simulink model "LineFollowerCar"  (R2022a)
settings: Solver=VariableStepAuto  StartTime=0.0  StopTime=10.0  RelTol=1e-3
libraries: arduinolib x8, simulink x3, slpidlib x1
settings Model: Creator=shuva  LastModifiedBy=shuva

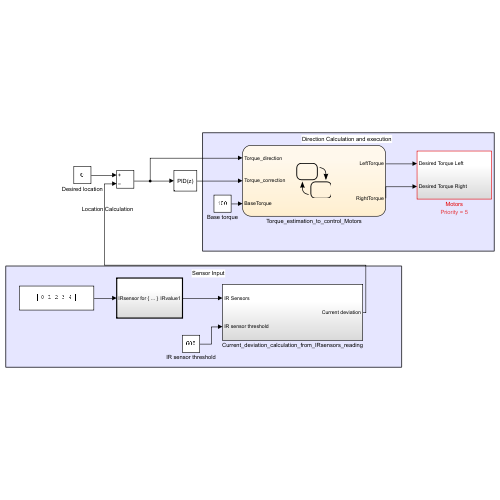
[thumbnail: Simulink's stored preview of the top-level diagram]
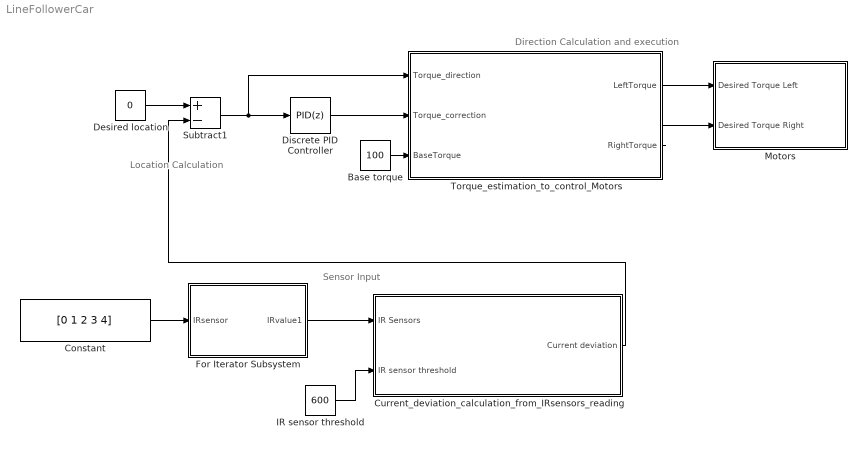
== system LineFollowerCar ==
  note: Sensor Input
  note: Direction Calculation and execution
  note: Location Calculation
  Base torque : Constant  Value=100  OutDataTypeStr=int16
  Constant : Constant  Value=[0 1 2 3 4]  OutDataTypeStr=uint8  SampleTime=0.002
  Current_deviation_calculation_from_IRsensors_reading : Subsystem
  Desired location : Constant  Value=0  OutDataTypeStr=int8
  Discrete PID Controller : slpidlib/PID Controller  Controller=PID  Form=Parallel  TimeDomain=Discrete-time  UseExternalTs=off  SampleTime=-1  IntegratorMethod=Forward Euler  FilterMethod=Forward Euler  ControllerParametersSource=internal  P=35  I=15  UseKiTs=off  D=0.005  N=60  UseFilter=off  TunerSelectOption=Transfer Function Based (PID Tuner App)  InitialConditionSource=internal  InitialConditionForIntegrator=0  InitialConditionForFilter=0  DifferentiatorICPrevScaledInput=0  ExternalReset=none  TrackingMode=off  Kt=1  LimitOutput=off  SatLimitsSource=internal  UpperSaturationLimit=inf  LowerSaturationLimit=-inf  LinearizeAsGain=on  AntiWindupMode=none  Kb=1  RndMeth=Round  PGainOutDataTypeStr=int16  PProdOutDataTypeStr=int16  POutMin=[]  POutMax=[]  IGainOutDataTypeStr=int16  IProdOutDataTypeStr=int16  IOutMin=[]  IOutMax=[]  DGainOutDataTypeStr=int16  DProdOutDataTypeStr=int16  DOutMin=[]  DOutMax=[]  NGainOutDataTypeStr=int8  NProdOutDataTypeStr=int8  NOutMin=[]  NOutMax=[]  SumOutDataTypeStr=int16  SumOutMin=[]  SumOutMax=[]  SaturationOutMin=[]  SaturationOutMax=[]  PParamDataTypeStr=int16  PParamMin=[]  PParamMax=[]  IParamDataTypeStr=int16  IParamMin=[]  IParamMax=[]  DParamDataTypeStr=int16  DParamMin=[]  DParamMax=[]  NParamDataTypeStr=int8  NParamMin=[]  NParamMax=[]  KbParamMin=[]  KbParamMax=[]  KtParamMin=[]  KtParamMax=[]  KbOutMin=[]  KbOutMax=[]  KtOutMin=[]  KtOutMax=[]  IntegratorOutDataTypeStr=int16  IntegratorOutMin=[]  IntegratorOutMax=[]  FilterOutDataTypeStr=int8  FilterOutMin=[]  FilterOutMax=[]  SumI1OutMin=[]  SumI1OutMax=[]  SumI2OutMin=[]  SumI2OutMax=[]  SumI3OutMin=[]  SumI3OutMax=[]  SumI4OutMin=[]  SumI4OutMax=[]  SumDOutDataTypeStr=int8  SumDOutMin=[]  SumDOutMax=[]  SumAccumDataTypeStr=int16  SumDAccumDataTypeStr=int8  DifferentiatorOutMin=[]  DifferentiatorOutMax=[]  FilterDiffOutCoefMin=[]  FilterDiffOutCoefMax=[]  ReciprocalOutMin=[]  ReciprocalOutMax=[]  SumDenOutMin=[]  SumDenOutMax=[]  SumNumOutMin=[]  SumNumOutMax=[]  DivideOutMin=[]  DivideOutMax=[]  UdiffTsProdOutMin=[]  UdiffTsProdOutMax=[]  NTsProdOutMin=[]  NTsProdOutMax=[]  UintegralTsProdOutMin=[]  UintegralTsProdOutMax=[]  UngainTsProdOutMin=[]  UngainTsProdOutMax=[]  IntegratorContinuousStateAttributes=''  IntegratorStateMustResolveToSignalObject=off  IntegratorRTWStateStorageClass=Auto  FilterContinuousStateAttributes=''  FilterStateMustResolveToSignalObject=off  FilterRTWStateStorageClass=Auto  ParallelPVariant=InternalParameters  IdealPVariant=Disabled  IVariant=InternalParameters  DVariant=InternalParameters  IntegratorVariant=Discrete  SatVariant=Disabled  AWVariant=Passthrough  PCopyVariant=Disabled  TRVariant=Disabled  FdbkBlocksVariant=Forward  IdealPFdbkVariant=Disabled  SatFdbkVariant=Disabled  DerivativeFilterVariant=Differentiator  NVariant=Passthrough  NCopyVariant=Disabled_SignalSpec  FilterICVariant=InternalICsDifferentiator  IntegratorICVariant=InternalICs  ExternalResetVariant=Disabled  TRSumVariant=Passthrough  SumFdbkVariant=Disabled  SumVariant=Sum_PID  TsampFilterVariant=InternalTs  TsampNgainVariant=Passthrough  TsampIntegralVariant=Passthrough  ExternalSaturationOutDataTypeStr=Inherit: Same as second input  aMode=0
  For Iterator Subsystem : Subsystem  TreatAsAtomicUnit=on
  IR sensor threshold : Constant  Value=600  OutDataTypeStr=int16
  Motors : Subsystem  Priority=5
      settings: AttributesFormatString=Priority = %<Priority>
  Subtract1 : Sum  Inputs=+-  AccumDataTypeStr=int8  OutDataTypeStr=int8
  Torque_estimation_to_control_Motors : Stateflow chart  TreatAsAtomicUnit=on
  wires:
  Subtract1/1 -> Torque_estimation_to_control_Motors/1(Torque_direction), Discrete PID Controller/1
  Desired location/1 -> Subtract1/1
  Base torque/1 -> Torque_estimation_to_control_Motors/3(BaseTorque)
  IR sensor threshold/1 -> Current_deviation_calculation_from_IRsensors_reading/2(IR sensor threshold)
  Constant/1 -> For Iterator Subsystem/1(IRsensor)
  For Iterator Subsystem/1(IRvalue1) -> Current_deviation_calculation_from_IRsensors_reading/1(IR Sensors)
  Current_deviation_calculation_from_IRsensors_reading/1(Current deviation) -> Subtract1/2
  Discrete PID Controller/1 -> Torque_estimation_to_control_Motors/2(Torque_correction)
  Torque_estimation_to_control_Motors/1(LeftTorque) -> Motors/1(Desired Torque Left)
  Torque_estimation_to_control_Motors/2(RightTorque) -> Motors/2(Desired Torque Right)

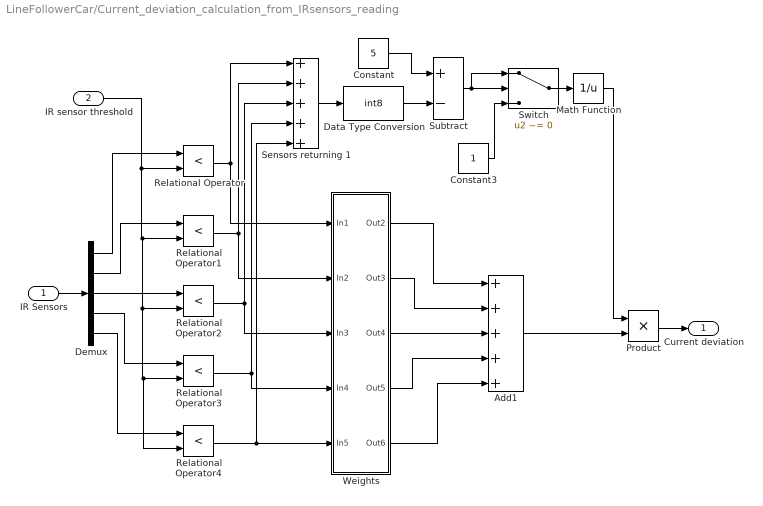
== system LineFollowerCar/Current_deviation_calculation_from_IRsensors_reading ==
  IR Sensors : Inport
  IR sensor threshold : Inport  Port=2
  Add1 : Sum  Inputs=+++++  AccumDataTypeStr=int8  OutDataTypeStr=int8
  Constant : Constant  Value=5  OutDataTypeStr=int8
  Constant3 : Constant  OutDataTypeStr=int8
  Data Type Conversion : DataTypeConversion  OutDataTypeStr=int8  SaturateOnIntegerOverflow=off  RndMeth=Floor
  Demux : Demux  Outputs=5
  Math Function : Math  Operator=reciprocal  SignedPower=on  OutDataTypeStr=Inherit: Inherit via internal rule
  Product : Product  OutDataTypeStr=int8  RndMeth=Round
  Relational Operator{,1..4} (5 alike) : RelationalOperator  Operator=<  OutDataTypeStr=boolean  InputSameDT=off
  Sensors returning 1 : Sum  Inputs=+++++  AccumDataTypeStr=int8  OutDataTypeStr=int8
  Subtract : Sum  Inputs=+-  AccumDataTypeStr=int8  OutDataTypeStr=int8  RndMeth=Round
  Switch : Switch  Criteria=u2 ~= 0  Threshold=0.0001  SaturateOnIntegerOverflow=off  InputSameDT=off
  Weights : Subsystem
  Current deviation : Outport  VectorParamsAs1DForOutWhenUnconnected=off
  wires:
  Math Function/1 -> Product/1
  Product/1 -> Current deviation/1
  Relational Operator/1 -> Weights/1(In1), Sensors returning 1/1
  Relational Operator1/1 -> Weights/2(In2), Sensors returning 1/2
  Relational Operator2/1 -> Sensors returning 1/3, Weights/3(In3)
  Relational Operator3/1 -> Sensors returning 1/4, Weights/4(In4)
  Relational Operator4/1 -> Sensors returning 1/5, Weights/5(In5)
  Add1/1 -> Product/2
  Weights/1(Out2) -> Add1/1
  Weights/3(Out4) -> Add1/3
  Weights/2(Out3) -> Add1/2
  Weights/4(Out5) -> Add1/4
  Weights/5(Out6) -> Add1/5
  Constant/1 -> Subtract/1
  Sensors returning 1/1 -> Data Type Conversion/1
  Demux/1 -> Relational Operator/1
  Demux/4 -> Relational Operator3/1
  Demux/5 -> Relational Operator4/1
  Demux/3 -> Relational Operator2/1
  Demux/2 -> Relational Operator1/1
  Subtract/1 -> Switch/1, Switch/2
  Switch/1 -> Math Function/1
  Constant3/1 -> Switch/3
  IR Sensors/1 -> Demux/1
  IR sensor threshold/1 -> Relational Operator4/2, Relational Operator3/2, Relational Operator2/2, Relational Operator1/2, Relational Operator/2
  Data Type Conversion/1 -> Subtract/2

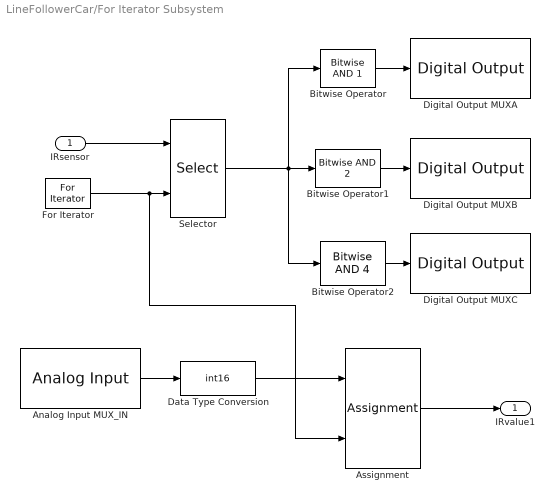
== system LineFollowerCar/For Iterator Subsystem ==
  IRsensor : Inport
  Analog Input MUX_IN : arduinolib/Analog Input  Priority=2  pinNumber=2  ReadResultsOnly=off  ConversionTriggerSource=Software  ExternalTriggerType=uint32(0)  OutputDataType=uint16  EnableConversionCompleteNotify=off  EnableOuputStatus=off  SampleTime=-1  blockPlatform=arduino
      settings: AttributesFormatString=Priority = %<Priority>
  Assignment : Assignment  IndexMode=Zero-based  OutputInitialize=Specify size for each dimension in table  DiagnosticForDimensions=Warning  IndexOptions=Index vector (port)  Indices=1  OutputSizes=5
  Bitwise Operator : simulink/Logic and Bit Operations/Bitwise Operator  logicop=AND  UseBitMask=on  BitMask=1  BitMaskRealWorld=Stored Integer
  Bitwise Operator1 : simulink/Logic and Bit Operations/Bitwise Operator  logicop=AND  UseBitMask=on  BitMask=2  BitMaskRealWorld=Stored Integer
  Bitwise Operator2 : simulink/Logic and Bit Operations/Bitwise Operator  logicop=AND  UseBitMask=on  BitMask=4  BitMaskRealWorld=Stored Integer
  Data Type Conversion : DataTypeConversion  OutDataTypeStr=int16  SaturateOnIntegerOverflow=off  RndMeth=Floor
  Digital Output MUXA : arduinolib/Digital Output  Priority=1  pinNumber=7  Direction=output  blockPlatform=arduino
      settings: AttributesFormatString=Priority = %<Priority>
  Digital Output MUXB : arduinolib/Digital Output  Priority=1  pinNumber=8  Direction=output  blockPlatform=arduino
      settings: AttributesFormatString=Priority = %<Priority>
  Digital Output MUXC : arduinolib/Digital Output  Priority=1  pinNumber=11  Direction=output  blockPlatform=arduino
      settings: AttributesFormatString=Priority = %<Priority>
  For Iterator : ForIterator  IndexMode=Zero-based  IterationVariableDataType=int8
  Selector : Selector  IndexMode=Zero-based  InputPortWidth=5  IndexOptions=Index vector (port)  Indices=[1 3]  OutputSizes=1
  IRvalue1 : Outport  VectorParamsAs1DForOutWhenUnconnected=off
  wires:
  For Iterator/1 -> Assignment/2, Selector/2
  IRsensor/1 -> Selector/1
  Selector/1 -> Bitwise Operator2/1, Bitwise Operator1/1, Bitwise Operator/1
  Bitwise Operator/1 -> Digital Output MUXA/1
  Bitwise Operator1/1 -> Digital Output MUXB/1
  Bitwise Operator2/1 -> Digital Output MUXC/1
  Analog Input MUX_IN/1 -> Data Type Conversion/1
  Assignment/1 -> IRvalue1/1
  Data Type Conversion/1 -> Assignment/1

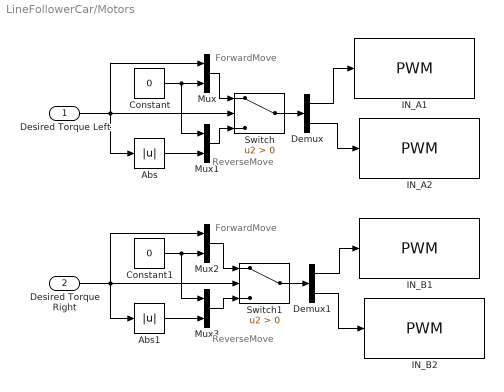
== system LineFollowerCar/Motors ==
  note: ReverseMove
  note: ForwardMove
  note: ReverseMove
  note: ForwardMove
  Desired Torque Left : Inport
  Desired Torque Right : Inport  Port=2
  Abs : Abs  OutDataTypeStr=int16  RndMeth=Round  SaturateOnIntegerOverflow=off
  Abs1 : Abs  OutDataTypeStr=int16  RndMeth=Round  SaturateOnIntegerOverflow=off
  Constant : Constant  Value=0  OutDataTypeStr=int16
  Constant1 : Constant  Value=0  OutDataTypeStr=int16
  Demux : Demux  Outputs=2
  Demux1 : Demux  Outputs=2
  IN_A1 : arduinolib/PWM  pinNumber=6  frequencyType=Default  desiredFrequency=490.2  achievableFrequency=490.2
  IN_A2 : arduinolib/PWM  pinNumber=5  frequencyType=Default  desiredFrequency=490.2  achievableFrequency=490.2
  IN_B1 : arduinolib/PWM  pinNumber=10  frequencyType=Default  desiredFrequency=490.2  achievableFrequency=490.2
  IN_B2 : arduinolib/PWM  pinNumber=9  frequencyType=Default  desiredFrequency=490.2  achievableFrequency=490.2
  Mux{,1..3} (4 alike) : Mux  Inputs=2
  Switch : Switch  Criteria=u2 > Threshold  SaturateOnIntegerOverflow=off  InputSameDT=off
  Switch1 : Switch  Criteria=u2 > Threshold  SaturateOnIntegerOverflow=off  InputSameDT=off
  wires:
  Desired Torque Left/1 -> Abs/1, Mux/1, Switch/2
  Switch/1 -> Demux/1
  Mux1/1 -> Switch/3
  Constant/1 -> Mux/2, Mux1/1
  Mux/1 -> Switch/1
  Abs/1 -> Mux1/2
  Desired Torque Right/1 -> Mux2/1, Abs1/1, Switch1/2
  Switch1/1 -> Demux1/1
  Mux3/1 -> Switch1/3
  Constant1/1 -> Mux2/2, Mux3/1
  Abs1/1 -> Mux3/2
  Demux1/1 -> IN_B1/1
  Demux/1 -> IN_A1/1
  Demux/2 -> IN_A2/1
  Demux1/2 -> IN_B2/1
  Mux2/1 -> Switch1/1

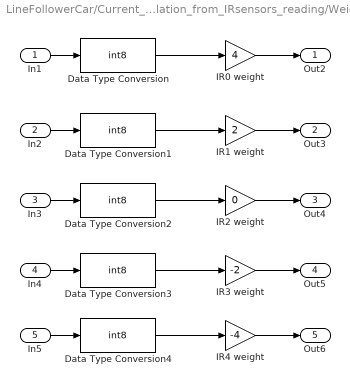
== system LineFollowerCar/Current_deviation_calculation_from_IRsensors_reading/Weights ==
  In1 : Inport
  In2 : Inport  Port=2
  In3 : Inport  Port=3
  In4 : Inport  Port=4
  In5 : Inport  Port=5
  Data Type Conversion{,1..4} (5 alike) : DataTypeConversion  OutDataTypeStr=int8  SaturateOnIntegerOverflow=off  RndMeth=Floor
  IR0 weight : Gain  Gain=4  OutDataTypeStr=int8
  IR1 weight : Gain  Gain=2  OutDataTypeStr=int8
  IR2 weight : Gain  Gain=0  OutDataTypeStr=int8
  IR3 weight : Gain  Gain=-2  OutDataTypeStr=int8
  IR4 weight : Gain  Gain=-4  OutDataTypeStr=int8
  Out2 : Outport  VectorParamsAs1DForOutWhenUnconnected=off
  Out3 : Outport  Port=2  VectorParamsAs1DForOutWhenUnconnected=off
  Out4 : Outport  Port=3  VectorParamsAs1DForOutWhenUnconnected=off
  Out5 : Outport  Port=4  VectorParamsAs1DForOutWhenUnconnected=off
  Out6 : Outport  Port=5  VectorParamsAs1DForOutWhenUnconnected=off
  wires:
  In2/1 -> Data Type Conversion1/1
  In1/1 -> Data Type Conversion/1
  In5/1 -> Data Type Conversion4/1
  In3/1 -> Data Type Conversion2/1
  In4/1 -> Data Type Conversion3/1
  IR0 weight/1 -> Out2/1
  IR2 weight/1 -> Out4/1
  IR1 weight/1 -> Out3/1
  IR3 weight/1 -> Out5/1
  IR4 weight/1 -> Out6/1
  Data Type Conversion3/1 -> IR3 weight/1
  Data Type Conversion4/1 -> IR4 weight/1
  Data Type Conversion2/1 -> IR2 weight/1
  Data Type Conversion1/1 -> IR1 weight/1
  Data Type Conversion/1 -> IR0 weight/1

== stateflow chart LineFollowerCar/Torque_estimation_to_control_Motors ==
  state GoStraight
    entry:
    LeftTorque = int16(15)+BaseTorque;
    RightTorque = int16(15)+BaseTorque;
  state TurnLeft
    entry:
    LeftTorque = BaseTorque - abs(Torque_correction);
    RightTorque = BaseTorque + abs(Torque_correction);
  state TurnRight
    entry:
    LeftTorque = BaseTorque + abs(Torque_correction);
    RightTorque = BaseTorque - abs(Torque_correction);
  (default) -> GoStraight
  GoStraight -> TurnRight [order 2] : [Torque_direction > 0]
  GoStraight -> TurnLeft [order 1] : [Torque_direction < 0]
  TurnRight -> GoStraight [order 1] : [Torque_direction == 0]
  TurnLeft -> GoStraight [order 2] : [Torque_direction == 0]
  TurnLeft -> TurnRight [order 1] : [Torque_direction > 0]
  TurnRight -> TurnLeft [order 2] : [Torque_direction < 0]
  data: Torque_direction input int8; Torque_correction input int16; BaseTorque input int16; LeftTorque output int16 [0..255]; RightTorque output int16 [0..255]
